simulink model "sgs_assin_2"  (R2025a)
settings: Solver=VariableStepAuto  StartTime=0.0  StopTime=2  RelTol=1e-3
libraries: spsIGBTDiodeLib x4, spsSeriesRLCBranchLib x4, spsVoltageMeasurementLib x3, spsCurrentMeasurementLib x2, simulink x2, spsACVoltageSourceLib x1, slpidlib x1, spsPLLLib x1, spsPVArrayLib x1, sps_lib x1
settings Model: Creator=bhargabgogoi  LastModifiedBy=bhargabgogoi

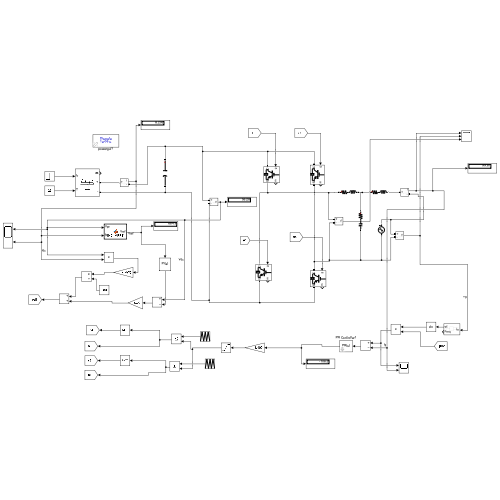
[thumbnail: Simulink's stored preview of the top-level diagram]
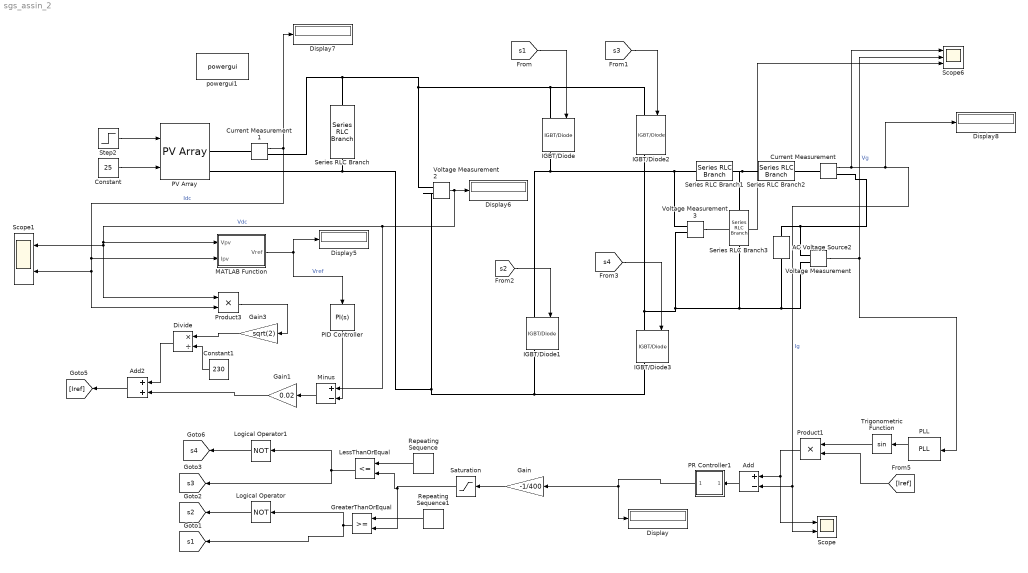
== system sgs_assin_2 ==
  AC Voltage Source2 : spsACVoltageSourceLib/AC Voltage Source  Amplitude=325  Phase=0  Frequency=50  SampleTime=0  Measurements=None  BusType=swing  Pref=10e3  Qref=0  Qmin=-inf  Qmax=+inf
  Add : Sum  Inputs=+-
  Add2 : Sum
  Constant : Constant  Value=25
  Constant1 : Constant  Value=230
  Current Measurement : spsCurrentMeasurementLib/Current Measurement  PhasorSimulation=off  OutputType=Complex  PSBequivalent=0
  Current Measurement1 : spsCurrentMeasurementLib/Current Measurement  PhasorSimulation=off  OutputType=Complex  PSBequivalent=0
  Display{,5..8} (5 alike) : Display
  Divide : Product  Inputs=*/
  Gain : Gain  Gain=-1/400
  Gain1 : Gain  Gain=0.02
  Gain3 : Gain  Gain=sqrt(2)
  GreaterThanOrEqual : RelationalOperator  OutDataTypeStr=boolean  RndMeth=Simplest  InputSameDT=off
  IGBT/Diode{,1..3} (4 alike) : spsIGBTDiodeLib/IGBT//Diode  Ron=1e-3  Rs=1e5  Cs=inf  Measurements=on
  LessThanOrEqual : RelationalOperator  Operator=<=  OutDataTypeStr=boolean  RndMeth=Simplest  InputSameDT=off
  Logical Operator : Logic  Operator=NOT  AllPortsSameDT=off  OutDataTypeStr=boolean
  Logical Operator1 : Logic  Operator=NOT  AllPortsSameDT=off  OutDataTypeStr=boolean
  MATLAB Function : MATLAB Function  TreatAsAtomicUnit=on
  Minus : Sum  Inputs=+-
  PID Controller : slpidlib/PID Controller  Controller=PI  Form=Parallel  TimeDomain=Continuous-time  UseExternalTs=off  SampleTime=-1  IntegratorMethod=Forward Euler  FilterMethod=Forward Euler  ControllerParametersSource=internal  P=0.3  I=0.1  UseKiTs=off  D=0  UseExternalDerivativeSource=off  N=100  UseFilter=on  TunerSelectOption=Transfer Function Based (PID Tuner App)  InitialConditionSource=internal  InitialConditionForIntegrator=0  InitialConditionForFilter=0  DifferentiatorICPrevScaledInput=0  ExternalReset=none  TrackingMode=off  Kt=1  LimitOutput=off  SatLimitsSource=internal  UpperSaturationLimit=inf  LowerSaturationLimit=-inf  LinearizeAsGain=on  AntiWindupMode=none  Kb=1  LimitIntegrator=off  UpperIntegratorSaturationLimit=inf  LowerIntegratorSaturationLimit=-inf  POutMin=[]  POutMax=[]  IOutMin=[]  IOutMax=[]  DOutMin=[]  DOutMax=[]  NOutMin=[]  NOutMax=[]  SumOutMin=[]  SumOutMax=[]  SaturationOutMin=[]  SaturationOutMax=[]  PParamMin=[]  PParamMax=[]  IParamMin=[]  IParamMax=[]  DParamMin=[]  DParamMax=[]  NParamMin=[]  NParamMax=[]  KbParamMin=[]  KbParamMax=[]  KtParamMin=[]  KtParamMax=[]  KbOutMin=[]  KbOutMax=[]  KtOutMin=[]  KtOutMax=[]  IntegratorOutMin=[]  IntegratorOutMax=[]  FilterOutMin=[]  FilterOutMax=[]  SumI1OutMin=[]  SumI1OutMax=[]  SumI2OutMin=[]  SumI2OutMax=[]  SumI3OutMin=[]  SumI3OutMax=[]  SumI4OutMin=[]  SumI4OutMax=[]  SumDOutMin=[]  SumDOutMax=[]  DifferentiatorOutMin=[]  DifferentiatorOutMax=[]  FilterDiffOutCoefMin=[]  FilterDiffOutCoefMax=[]  ReciprocalOutMin=[]  ReciprocalOutMax=[]  SumDenOutMin=[]  SumDenOutMax=[]  SumNumOutMin=[]  SumNumOutMax=[]  DivideOutMin=[]  DivideOutMax=[]  UdiffTsProdOutMin=[]  UdiffTsProdOutMax=[]  NTsProdOutMin=[]  NTsProdOutMax=[]  UintegralTsProdOutMin=[]  UintegralTsProdOutMax=[]  UngainTsProdOutMin=[]  UngainTsProdOutMax=[]  ClampingZeroOutDataTypeStr=Inherit: Inherit via back propagation  ClampingZeroOutMin=[]  ClampingZeroOutMax=[]  FilterDenConstantOutDataTypeStr=Inherit: Inherit via back propagation  FilterDenConstantOutMin=[]  FilterDenConstantOutMax=[]  PCopyOutDataTypeStr=Inherit: Inherit via back propagation  PCopyOutMin=[]  PCopyOutMax=[]  NCopyOutDataTypeStr=Inherit: Inherit via back propagation  NCopyOutMin=[]  NCopyOutMax=[]  IntegratorContinuousStateAttributes=''  IntegratorStateMustResolveToSignalObject=off  IntegratorRTWStateStorageClass=Auto  FilterContinuousStateAttributes=''  FilterStateMustResolveToSignalObject=off  FilterRTWStateStorageClass=Auto  ParallelPVariant=InternalParameters  IdealPVariant=Disabled  IVariant=InternalParameters  DVariant=Disabled  IntegratorVariant=Continuous  SatVariant=Disabled  AWVariant=Passthrough  PCopyVariant=Disabled  TRVariant=Disabled  FdbkBlocksVariant=Forward  IdealPFdbkVariant=Disabled  SatFdbkVariant=Disabled  DerivativeFilterVariant=Disabled  NVariant=Disabled  NCopyVariant=Disabled_SignalSpec  FilterICVariant=Disabled  IntegratorICVariant=InternalICs  ExternalResetVariant=Disabled  TRSumVariant=Passthrough  SumFdbkVariant=Disabled  SumVariant=Sum_PI  TsampFilterVariant=InternalTs  TsampNgainVariant=Passthrough  TsampIntegralVariant=Disabled_SignalSpec  ExternalSaturationOutDataTypeStr=Inherit: Same as second input  DerivativeSourceVariant=Disabled  PreIntVariant=InternalPreInt
  PLL : spsPLLLib/PLL  Fmin=45  Par_Init=[0, 50]  ParK=[180, 3200, 1]  TcD=1e-4  MaxRateChangeFreq=12  FilterCutOffFreq=25  Ts=0  AGC=on
      settings: LibrarySourceBlock=sps_lib/Control/PLL
  PR Controller1 : Subsystem  mask(PR Controller){kp=1.2, kr=750, f=50}
      mask prompts: kp "Proportional Gain (kp)"; kr "Resonant Gain (kr)"; f "Resonant Frequency (Hz)"
      mask help:
      | This block implements a Proportional Resonant Controller using transfer function kr*s / s^2+(2*pi*f)^2
      | It allows user to set the proportional gain (kp), resonant gain (kr) and resonant frequency in (Hz).
      |
      | Developed by Rodney Tan
      | Version 1.0 (Oct 2022)
      mask Display: disp('PR(s)');
  PV Array : spsPVArrayLib/PV Array  Npar=1  Nser=12  PlotType=array @ 1000 W/m2 & specified temperatures  S_vec="[ 1000  500  100 ]"  Temp_C_vec="[ 45 25  ]"  ModuleName=User-defined  PlotWhenSelected=off  Pm=235.008  Ncell=60  Voc=36.72  Isc=8.23  Vm=30.6  Im=7.68  beta_Voc_pc=-0.359  alpha_Isc_pc=0.096999  beta_Voc=-0.13182  alpha_Isc=0.007983  IL=8.2383  I0=2.8334e-10  nI=0.98962  Rsh=196.9274  Rs=0.19811  RobustModel=off  RobustCellTemperature=313.3991  BAL=on  Tc=1e-6  Tfilter=5e-5
  Product1 : Product
  Product3 : Product
  Repeating Sequence : simulink/Sources/Repeating Sequence  rep_seq_t=[0 1/10000 1/5000]  rep_seq_y=[-1 0 -1]
  Repeating Sequence1 : simulink/Sources/Repeating Sequence  rep_seq_t=[0 1/10000 1/5000]  rep_seq_y=[0 1 0 ]
  Saturation : Saturate  UpperLimit=1  LowerLimit=-1
  Scope : Scope  NumInputPorts=2
      settings: ActiveDisplayYMinimum=-25.492308794050363  ActiveDisplayYMaximum=25.49696496406396
  Scope1 : Scope  NumInputPorts=2
      settings: ActiveDisplayYMinimum=389.53599855540983  ActiveDisplayYMaximum=547.36305056852018
  Scope6 : Scope  NumInputPorts=3
      settings: ActiveDisplayYMinimum=-338.17620680157967  ActiveDisplayYMaximum=340.0158999737796  DataLoggingVariableName=ScopeData6
  Series RLC Branch : spsSeriesRLCBranchLib/Series RLC Branch  LConnTagsString=__new0  RConnTagsString=__new0  BranchType=C  Resistance=0.01  Inductance=1e-3  SetiL0=off  InitialCurrent=0  Capacitance=1000e-6  Setx0=on  InitialVoltage=500  Measurements=None
  Series RLC Branch1 : spsSeriesRLCBranchLib/Series RLC Branch  LConnTagsString=__new0  RConnTagsString=__new0  BranchType=RL  Resistance=0.001  Inductance=6e-3  SetiL0=off  InitialCurrent=0  Capacitance=1e-6  Setx0=off  InitialVoltage=0  Measurements=None
  Series RLC Branch2 : spsSeriesRLCBranchLib/Series RLC Branch  LConnTagsString=__new0  RConnTagsString=__new0  BranchType=RL  Resistance=0.001  Inductance=6e-3  SetiL0=off  InitialCurrent=0  Capacitance=1e-6  Setx0=off  InitialVoltage=0  Measurements=None
  Series RLC Branch3 : spsSeriesRLCBranchLib/Series RLC Branch  LConnTagsString=__new0  RConnTagsString=__new0  BranchType=RC  Resistance=0.001  Inductance=70e-3  SetiL0=off  InitialCurrent=0  Capacitance=0.2e-6  Setx0=off  InitialVoltage=0  Measurements=None
  Step2 : Step  Time=0.5  Before=500  After=1000  SampleTime=0
  Trigonometric Function : Trigonometry
  Voltage Measurement : spsVoltageMeasurementLib/Voltage Measurement  PhasorSimulation=off  OutputType=Complex  PSBequivalent=0
  Voltage Measurement2 : spsVoltageMeasurementLib/Voltage Measurement  PhasorSimulation=off  OutputType=Complex  PSBequivalent=0
  Voltage Measurement3 : spsVoltageMeasurementLib/Voltage Measurement  PhasorSimulation=off  OutputType=Complex  PSBequivalent=0
  powergui1 : sps_lib/powergui  Priority=1  SimulationMode=Discrete  SampleTime=1e-6  frequency=60  Iterations=50  frequencyindice=0  Pbase=100e6  ErrMax=1e-4  UnitsV=kV  UnitsW=MW  buscounter=0  FunctionMessages=off  echomessages=off  EnableUseOfTLC=off  CurrentSourceSwitches=off  DisableSnubberDevices=off  DisableRonSwitches=off  DisableVfSwitches=off  DisplayEquations=off  AutomaticDiscreteSolvers=off  SolverType=Tustin/Backward Euler (TBE)  Interpol=off  ExternalGateDelay=off  methode=off  Ts=100  x0status=blocks  SPID=on  SwTol=0  HookPort=off  NonlinearTolerance=1e-4  nMaxIteration=100  ContinueOnMaxIteration=off  RestoreLinks=warning  ResistiveCurrentMeasurement=off  Frange=[0:2:500]  Ylog=off  Xlog=on  ShowGrid=off  save=off  variable=ZData  structure=0  ZoomFFT=off  StartTime=0.0  cycles=1  DisplayStyle=1  fundamental=60  FreqAxis=off  MaxFrequency=1000  frequencyindicesteady=1  RmsSteady=1  display=off
  tag scope: s1=global, s2=global, s3=global, s4=global
  wires:
  [Iref] -> Product1/2
  Current Measurement/1 -> Scope6/1, Display8/1, Scope/2, Add/2  "Ig"
  Trigonometric Function/1 -> Product1/1
  Voltage Measurement/1 -> Scope6/2, PLL/1  "Vg"
  Step2/1 -> PV Array/1
  Product3/1 -> Gain3/1
  Constant/1 -> PV Array/2
  Current Measurement1/1 -> Display7/1, Product3/2, Scope1/2, MATLAB Function/2(Ipv)  "Idc"
  Minus/1 -> Gain1/1
  Gain3/1 -> Divide/1
  Gain1/1 -> Add2/2
  Divide/1 -> Add2/1
  Add2/1 -> [Iref]
  Product1/1 -> Scope/1, Add/1
  LessThanOrEqual/1 -> [s3], Logical Operator1/1
  Logical Operator1/1 -> [s4]
  Repeating Sequence1/1 -> GreaterThanOrEqual/1
  Saturation/1 -> GreaterThanOrEqual/2, LessThanOrEqual/2
  Repeating Sequence/1 -> LessThanOrEqual/1
  Voltage Measurement2/1 -> Display6/1, Minus/1, Product3/1, Scope1/1, MATLAB Function/1(Vpv)  "Vdc"
  GreaterThanOrEqual/1 -> [s1], Logical Operator/1
  Logical Operator/1 -> [s2]
  PLL/2 -> Trigonometric Function/1
  Constant1/1 -> Divide/2
  [s1] -> IGBT/Diode/1
  [s3] -> IGBT/Diode2/1
  [s2] -> IGBT/Diode1/1
  [s4] -> IGBT/Diode3/1
  Voltage Measurement3/1 -> Scope6/3
  Add/1 -> PR Controller1/1(In1)
  Gain/1 -> Saturation/1
  PR Controller1/1(Out1) -> Gain/1, Display/1
  PID Controller/1 -> Minus/2
  MATLAB Function/1(Vref) -> Display5/1, PID Controller/1  "Vref"
  connections:
  Voltage Measurement/LConn2 -- IGBT/Diode2/RConn1 -- IGBT/Diode3/LConn1 -- Voltage Measurement3/LConn2 -- Series RLC Branch3/RConn1 -- AC Voltage Source2/LConn1
  Series RLC Branch/LConn1 -- Current Measurement1/RConn1 -- Voltage Measurement2/LConn1 -- IGBT/Diode/LConn1 -- IGBT/Diode2/LConn1
  IGBT/Diode1/LConn1 -- Voltage Measurement3/LConn1 -- Series RLC Branch1/LConn1 -- IGBT/Diode/RConn1
  Voltage Measurement2/LConn2 -- IGBT/Diode3/RConn1 -- IGBT/Diode1/RConn1 -- Series RLC Branch/RConn1 -- PV Array/RConn2
  PV Array/RConn1 -- Current Measurement1/LConn1
  AC Voltage Source2/RConn1 -- Current Measurement/RConn1 -- Voltage Measurement/LConn1
  Series RLC Branch2/LConn1 -- Series RLC Branch3/LConn1 -- Series RLC Branch1/RConn1
  Series RLC Branch2/RConn1 -- Current Measurement/LConn1

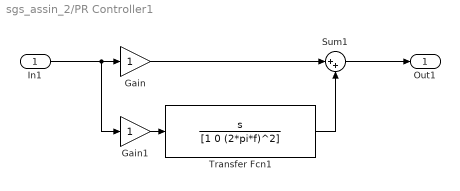
== system sgs_assin_2/PR Controller1 ==
  In1 : Inport
  Gain : Gain
  Gain1 : Gain
  Sum1 : Sum  Inputs=|++
  Transfer Fcn1 : TransferFcn  Numerator=[1 0]  Denominator=[1 0 (2*pi*f)^2]
  Out1 : Outport
  wires:
  Gain1/1 -> Transfer Fcn1/1
  Transfer Fcn1/1 -> Sum1/2
  In1/1 -> Gain1/1, Gain/1
  Sum1/1 -> Out1/1
  Gain/1 -> Sum1/1

== matlab function sgs_assin_2/MATLAB Function ==
  data: Vpv input; Vref output; Ipv input
function Vref = INC_MPPT(Vpv, Ipv)
%%#codegen
% Incremental Conductance MPPT
% Input : PV voltage and PV current
% Output: DC-link/PV voltage reference

persistent Vprev Iprev Vref_prev

if isempty(Vprev)
    Vprev = Vpv;
    Iprev = Ipv;
    Vref_prev = Vpv;
end

% MPPT voltage step
DeltaVref = 0.0002;

% Tolerance
eps_val = 1e-6;

% Changes in PV voltage and current
dV = Vpv - Vprev;
dI = Ipv - Iprev;

if abs(dV) < eps_val

    if abs(dI) < eps_val
        % At MPP
        Vref = Vref_prev;

    elseif dI > 0
        % Move toward higher voltage
        Vref = Vref_prev + DeltaVref;

    else
        % Move toward lower voltage
        Vref = Vref_prev - DeltaVref;
    end

else

    % Incremental conductance
    IncCond = dI / dV;

    % Instantaneous conductance
    InstCond = -Ipv / Vpv;

    if abs(IncCond - InstCond) < eps_val
        % At MPP
        Vref = Vref_prev;

    elseif IncCond > InstCond
        % Left of MPP
        Vref = Vref_prev + DeltaVref;

    else
        % Right of MPP
        Vref = Vref_prev - DeltaVref;
    end
end

% Update previous values
Vprev = Vpv;
Iprev = Ipv;
Vref_prev = Vref;

end
